simulink model "nabludatelSimulink"  (Simulink 7.8)
settings: Solver=ode45  StartTime=0.0  StopTime=10.0  RelTol=1e-3
values from neighbouring files (symbols this model uses):
  C = get(gca, 'CurrentPoint')    [movecirc.m]    (also in plotcurv2.m; plotcurve.m = get(gca,'CurrentPoint'))
undefined symbols (not defined in the file or in its folder): A, B
settings Model: Creator=--  LastModifiedBy=--

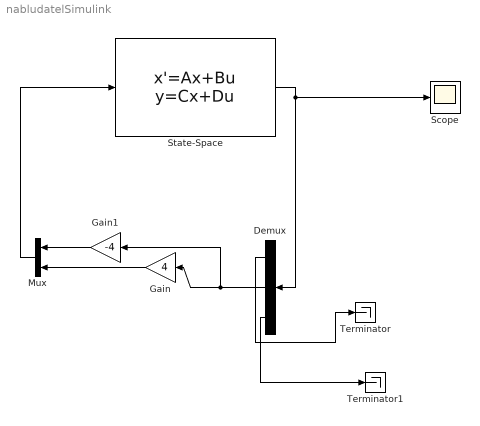
== system nabludatelSimulink ==
  Demux : Demux  Outputs=3
  Gain : Gain  Gain=4
  Gain1 : Gain  Gain=-4
  Mux : Mux  Inputs=2
  Scope : Scope
  State-Space : StateSpace  A=A  B=B  C=C  D=[0 0 ; 0 0; 0 0]  X0=[1 2 3]'
  Terminator : Terminator
  Terminator1 : Terminator
  wires:
  State-Space/1 -> Demux/1, Scope/1
  Gain/1 -> Mux/2
  Gain1/1 -> Mux/1
  Mux/1 -> State-Space/1
  Demux/1 -> Terminator/1
  Demux/3 -> Terminator1/1
  Demux/2 -> Gain/1, Gain1/1
